simulink model "calculate_intersection"  (R2018a)
settings: Solver=VariableStepAuto  StartTime=0.0  StopTime=10.0  RelTol=1e-3
libraries: simulink x3
settings Model: Creator=blond  LastModifiedBy=blond

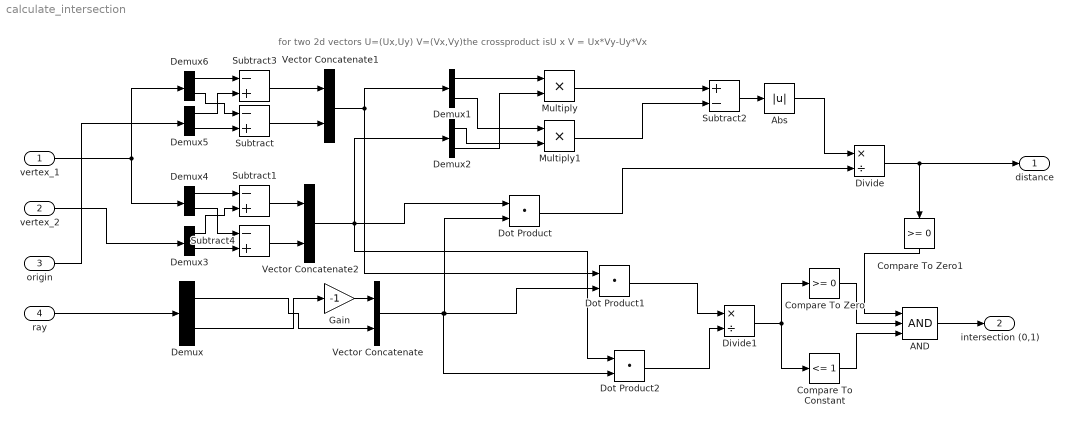
== system calculate_intersection ==
  note: for two 2d vectors U=(Ux,Uy) V=(Vx,Vy)the crossproduct isU x V = Ux*Vy-Uy*Vx
  vertex_1 : Inport
  vertex_2 : Inport  Port=2
  "origin " : Inport  Port=3
  ray : Inport  Port=4
  AND : Logic  Inputs=3  IconShape=distinctive  AllPortsSameDT=off  OutDataTypeStr=boolean
  Abs : Abs  ZeroCross=off
  Compare To Constant : simulink/Logic and Bit Operations/Compare To Constant  relop=<=  const=1  OutDataTypeStr=boolean  ZeroCross=off
  Compare To Zero : simulink/Logic and Bit Operations/Compare To Zero  relop=>=  OutDataTypeStr=boolean  ZeroCross=off
  Compare To Zero1 : simulink/Logic and Bit Operations/Compare To Zero  relop=>=  OutDataTypeStr=boolean  ZeroCross=off
  Demux{,1..6} (7 alike) : Demux  Outputs=2
  Divide : Product  Inputs=*/
  Divide1 : Product  Inputs=*/
  Dot Product : DotProduct  InputSameDT=on  OutDataTypeStr=Inherit: Inherit via internal rule
  Dot Product1 : DotProduct  InputSameDT=on  OutDataTypeStr=Inherit: Inherit via internal rule
  Dot Product2 : DotProduct  InputSameDT=on  OutDataTypeStr=Inherit: Inherit via internal rule
  Gain : Gain  Gain=-1
  Multiply : Product
  Multiply1 : Product
  Subtract{,1,3..4} (4 alike) : Sum  Inputs=-+
  Subtract2 : Sum  Inputs=+-
  Vector Concatenate : Concatenate
  Vector Concatenate1 : Concatenate
  Vector Concatenate2 : Concatenate
  distance : Outport
  intersection (0,1) : Outport  Port=2
  wires:
  Dot Product1/1 -> Divide1/1
  Abs/1 -> Divide/1
  Subtract2/1 -> Abs/1
  Demux1/2 -> Multiply1/1
  Multiply/1 -> Subtract2/1
  Gain/1 -> Vector Concatenate/1
  Subtract4/1 -> Vector Concatenate2/2
  Dot Product/1 -> Divide/2
  ray/1 -> Demux/1
  Compare To Zero/1 -> AND/2
  Vector Concatenate2/1 -> Dot Product/1, Demux2/1, Dot Product2/1
  vertex_1/1 -> Demux6/1, Demux4/1
  Dot Product2/1 -> Divide1/2
  Vector Concatenate1/1 -> Dot Product1/1, Demux1/1
  Demux2/1 -> Multiply1/2
  Demux4/2 -> Subtract4/1
  Demux3/1 -> Subtract1/2
  Compare To Zero1/1 -> AND/1
  Vector Concatenate/1 -> Dot Product/2, Dot Product1/2, Dot Product2/2
  Divide1/1 -> Compare To Zero/1, Compare To Constant/1
  Multiply1/1 -> Subtract2/2
  AND/1 -> intersection (0,1)/1
  Demux3/2 -> Subtract4/2
  Demux5/2 -> Subtract/2
  Demux6/2 -> Subtract/1
  Demux4/1 -> Subtract1/1
  Demux2/2 -> Multiply/2
  Demux5/1 -> Subtract3/2
  Subtract3/1 -> Vector Concatenate1/1
  vertex_2/1 -> Demux3/1
  "origin "/1 -> Demux5/1
  Divide/1 -> distance/1, Compare To Zero1/1
  Demux6/1 -> Subtract3/1
  Subtract1/1 -> Vector Concatenate2/1
  Demux1/1 -> Multiply/1
  Subtract/1 -> Vector Concatenate1/2
  Compare To Constant/1 -> AND/3
  Demux/1 -> Vector Concatenate/2
  Demux/2 -> Gain/1
